simulink model "SimulinkModel_OWC_Array_Generator_Control_Varying_Theta"  (R2017b)
settings: Solver=ode4  StartTime=0.0  StopTime=tsim  FixedStep=delta_t  RelTol=1e-3
values from neighbouring files (symbols this model uses):
  a_gen = 0.0001    [InputDataExtraction.m]
  activate_HSSV = 1    [InputDataExtraction.m]
  Ainf_inv = inv(Ainf)    [InputDataExtraction.m]
  alpha1 = 219.4    [InputDataExtraction.m]
  alpha2 = 219.54    [InputDataExtraction.m]
  alpha3 = 219.4    [InputDataExtraction.m]
  B = zeros(vz,hz)    [ACTOR_CRITIC & SARSA.m]    (also in InputDataExtraction.m = 0.01; TDlearningExampleEforPosting.m)
  b_gen = 3.6    [InputDataExtraction.m]
  Beta = 30    [InputDataExtraction.m]
  d_t = 0.5    [InputDataExtraction.m]
  FEX = squeeze(FEX_ma_temp(:,ind_w-1+step)- ((omega -FEX_Sim.Omega(ind_w-1))/(FEX_Sim.Omega(ind_w)-FEX_Sim.Omega(ind_w-1))*(FEX_ma_temp(:,ind_w+step)-FEX_ma_temp(:,ind_w-1+step))))    [InputDataExtraction.m]
  FEX_ph = FEX_ph.*pi./180    [InputDataExtraction.m]
  gamma = 0.1    [CS533DQN_FunctionApproximation.m]    (also in ContinousControl.m = 0.75; DeepQLearningF.m = 0.25; HopeGreatRLCode.m = 0.3; InputDataExtraction.m = 1.4)
  h_zero = 15    [InputDataExtraction.m]
  Height = states_space(next_stPrimee_idx,1)    [ContinousControl.m]    (also in DeepQLearningF.m = states_space(state_idx,1); EtanStateExtraction.m = HeightVec(h); Forward_step.m = states_space( st_chosen,1); InputDataExtraction.m = HeightVec(h))
  I_c = [0 ... (first row only)    [InputDataExtraction.m]
  I_c_kin = [55 ... (first row only)    [InputDataExtraction.m]
  I_c_turb = [0 ... (first row only)    [InputDataExtraction.m]
  i_ms = 1.7    [InputDataExtraction.m]
  J = 3.06    [InputDataExtraction.m]
  K_buoancy = diag([ -rho*g*(S_b-S_p) -rho*g*(S_b-S_p) -rho*g*(S_b-S_p) -rho*g*S_p -rho*g*S_p -rho*g*S_p])    [InputDataExtraction.m]
  K_mooring = diag([K_m K_m K_m 0 0 0])    [InputDataExtraction.m]
  K_pressure = [ p_at*S_p p_at*S_p p_at*S_p]    [InputDataExtraction.m]
  L_m = 7.413    [InputDataExtraction.m]
  L_s = 0.13    [InputDataExtraction.m]
  Nt = 2    [InputDataExtraction.m]
  omega = (2*pi)/Ts    (= 0.628318530718)    [InputDataExtraction.m]
  OmegaStar = 6000/60    (= 100)    [InputDataExtraction.m]
  p_at = 1.01325*10e5    (= 1013250)    [InputDataExtraction.m]
  poles = 2    [InputDataExtraction.m]
  rho_at = 1.2041    [InputDataExtraction.m]
  s1 = 0.11    [InputDataExtraction.m]
  s2 = 0.11    [InputDataExtraction.m]
  s3 = 0.11    [InputDataExtraction.m]
  S_p = (d_p/2)^2*pi    (= 15.7632552987)    [InputDataExtraction.m]
  T_loss = 3    [InputDataExtraction.m]
  time_shift = -min(FEX_ph*Tp)*ones(6,1)    [InputDataExtraction.m]
  Tp = Ts    (= 10)    [InputDataExtraction.m]    (also in LetsStartIt.m = Ts; SafeLetsStartIt.m = Ts; StateExtraction.m = Ts)
  wave_delay = [wave_delay; wave_delay]    [InputDataExtraction.m]
undefined symbols (not defined in the file or in its folder): A_SS_R, B_SS_R, C_SS_R, D_SS_R
settings Model: Creator=danie  LastModifiedBy=browdani
settings OptimizationCC: LifeSpan=inf
settings DebuggingCC: SFExecutionAtInitializationDiag=none
settings CodeAppCC: StateflowObjectComments=on

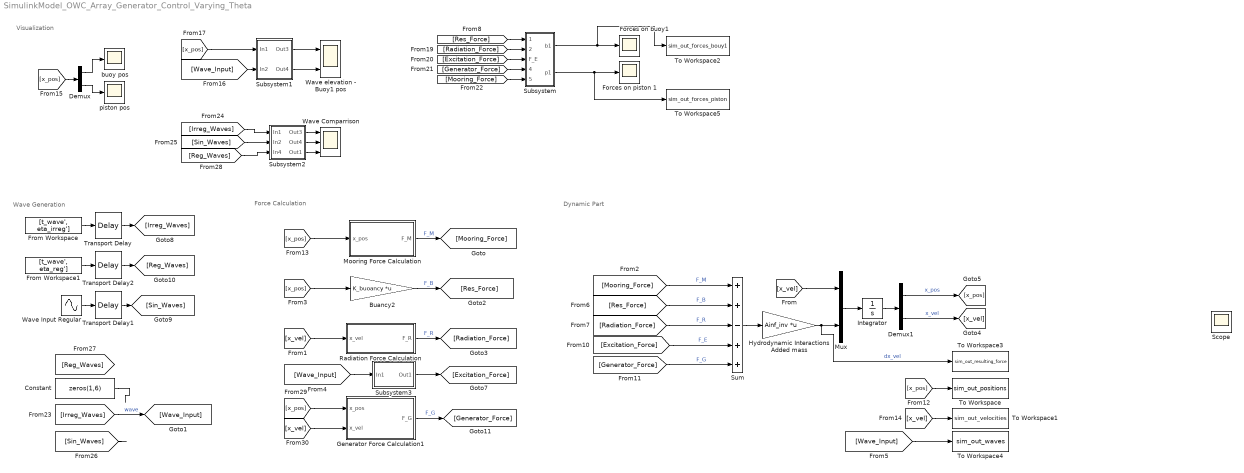
== system SimulinkModel_OWC_Array_Generator_Control_Varying_Theta ==
  note: Wave Generation
  note: Force Calculation
  note: Visualization
  note: Dynamic Part
  Buancy2 : Gain  Gain=K_buoancy  Multiplication=Matrix(K*u)
  Constant : Constant  Value=zeros(1,6)
  Demux : Demux  Outputs=2
  Demux1 : Demux  Outputs=2
  "Forces on buoy1 " : Scope
  Forces on piston 1 : Scope
  From Workspace : FromWorkspace  VariableName=[t_wave', eta_irreg']  SampleTime=0
  From Workspace1 : FromWorkspace  VariableName=[t_wave', eta_reg']  SampleTime=0
  Generator Force Calculation1 : Subsystem
  Hydrodynamic Interactions Added mass : Gain  Gain=Ainf_inv  Multiplication=Matrix(K*u)
  Integrator : Integrator  InitialCondition=I_c
  "Mooring Force Calculation " : Subsystem
  Mux : Mux  Inputs=2
  Radiation Force Calculation : Subsystem
  Subsystem : Subsystem
  Subsystem1 : Subsystem
  Subsystem2 : Subsystem
  Subsystem3 : Subsystem
  Sum : Sum  Inputs=++-++
  To Workspace : ToWorkspace  VariableName=sim_out_positions  SampleTime=-1
  To Workspace1 : ToWorkspace  VariableName=sim_out_velocities  SampleTime=-1
  To Workspace2 : ToWorkspace  VariableName=sim_out_forces_bouy1  SampleTime=-1
  To Workspace3 : ToWorkspace  VariableName=sim_out_resulting_force  SampleTime=-1
  To Workspace4 : ToWorkspace  VariableName=sim_out_waves  SampleTime=-1
  To Workspace5 : ToWorkspace  VariableName=sim_out_forces_piston  SampleTime=-1
  Transport Delay : TransportDelay  DelayTime=wave_delay +(time_shift+FEX_ph*Tp)
  Transport Delay1 : TransportDelay  DelayTime=wave_delay +(time_shift+FEX_ph*Tp)
  Transport Delay2 : TransportDelay  DelayTime=wave_delay +(time_shift+FEX_ph*Tp)
  Wave Comparrison : Scope  NumInputPorts=3
  Wave Input Regular : Sin  Amplitude=Height/2  Frequency=omega  Phase=FEX_ph  SampleTime=0
  "Wave elevation - Buoy1 pos " : Scope  NumInputPorts=2
  "buoy pos " : Scope
  "piston pos " : Scope
  Scope : Scope
  wires:
  [x_vel] -> Radiation Force Calculation/1(x_vel)
  Sum/1 -> Hydrodynamic Interactions Added mass/1
  Demux1/2 -> [x_vel]  "x_vel"
  Demux1/1 -> [x_pos]  "x_pos"
  Hydrodynamic Interactions Added mass/1 -> To Workspace3/1, Mux/2  "dx_vel"
  Subsystem/1(b1) -> To Workspace2/1, "Forces on buoy1 "/1
  Subsystem/2(p1) -> To Workspace5/1, Forces on piston 1/1
  [x_pos] -> "Mooring Force Calculation "/1(x_pos)
  [Generator_Force] -> Sum/5  "F_G"
  Subsystem1/1(Out3) -> "Wave elevation - Buoy1 pos "/1
  Subsystem1/2(Out4) -> "Wave elevation - Buoy1 pos "/2
  [Res_Force] -> Sum/2  "F_B"
  "Mooring Force Calculation "/1(F_M) -> [Mooring_Force]  "F_M"
  [Mooring_Force] -> Sum/1  "F_M"
  [Wave_Input] -> Subsystem3/1(In1)
  [x_pos] -> Buancy2/1
  Buancy2/1 -> [Res_Force]  "F_B"
  Radiation Force Calculation/1(F_R) -> [Radiation_Force]  "F_R"
  [Radiation_Force] -> Sum/3  "F_R"
  [Excitation_Force] -> Sum/4  "F_E"
  [x_pos] -> To Workspace/1
  [x_vel] -> To Workspace1/1
  [x_pos] -> Demux/1
  Demux/1 -> "buoy pos "/1
  Demux/2 -> "piston pos "/1
  [Wave_Input] -> Subsystem1/2(In2)
  [x_pos] -> Subsystem1/1(In1)
  [Res_Force] -> Subsystem/1(F_B)
  [Radiation_Force] -> Subsystem/2(F_R)
  [Excitation_Force] -> Subsystem/3(F_E)
  [Generator_Force] -> Subsystem/4(F_G)
  [Mooring_Force] -> Subsystem/5(F_M)
  Wave Input Regular/1 -> Transport Delay1/1
  [Irreg_Waves] -> Subsystem2/1(In1)
  [Sin_Waves] -> Subsystem2/2(In2)
  [Sin_Waves] -> ?
  Constant/1 -> ?
  From Workspace/1 -> Transport Delay/1
  Transport Delay/1 -> [Irreg_Waves]
  Transport Delay1/1 -> [Sin_Waves]
  Transport Delay2/1 -> [Reg_Waves]
  From Workspace1/1 -> Transport Delay2/1
  [Reg_Waves] -> Subsystem2/3(In4)
  Generator Force Calculation1/1(F_G) -> [Generator_Force]  "F_G"
  [x_vel] -> Generator Force Calculation1/2(x_vel)
  [x_pos] -> Generator Force Calculation1/1("x_pos ")
  [x_vel] -> Mux/1
  Mux/1 -> Integrator/1
  Integrator/1 -> Demux1/1
  Subsystem2/1(Out3) -> Wave Comparrison/1
  Subsystem2/2(Out4) -> Wave Comparrison/2
  Subsystem2/3(Out1) -> Wave Comparrison/3
  Subsystem3/1(Out1) -> [Excitation_Force]
  [Wave_Input] -> To Workspace4/1
  [Irreg_Waves] -> [Wave_Input]  "wave"

== system SimulinkModel_OWC_Array_Generator_Control_Varying_Theta/Generator Force Calculation1 ==
  "x_pos " : Inport
  x_vel : Inport  Port=2
  Gain : Gain  Gain=K_pressure
  Gain1 : Gain  Gain=-K_pressure
  Mux3 : Mux  Inputs=2
  To Workspace : ToWorkspace  VariableName=sim_out_chamber_pressure  SampleTime=-1
  Turbine/Generator Dynamics : Subsystem
  F_G : Outport
  wires:
  "x_pos "/1 -> Turbine/Generator Dynamics/1(x_pos)
  x_vel/1 -> Turbine/Generator Dynamics/2("x_vel ")
  Turbine/Generator Dynamics/1("p* ") -> Gain/1, Gain1/1, To Workspace/1
  Mux3/1 -> F_G/1  "F_G"
  Gain1/1 -> Mux3/2
  Gain/1 -> Mux3/1

== system SimulinkModel_OWC_Array_Generator_Control_Varying_Theta/Mooring Force Calculation  ==
  x_pos : Inport
  Buancy1 : Gain  Gain=K_mooring  Multiplication=Matrix(K*u)
  Constant : Constant  Value=0
  "Only if heave coordinte >0, extension of cables" : MinMax  Function=max  Inputs=2
  F_M : Outport
  wires:
  Constant/1 -> "Only if heave coordinte >0, extension of cables"/2
  Buancy1/1 -> F_M/1  "F_M"
  x_pos/1 -> "Only if heave coordinte >0, extension of cables"/1
  "Only if heave coordinte >0, extension of cables"/1 -> Buancy1/1

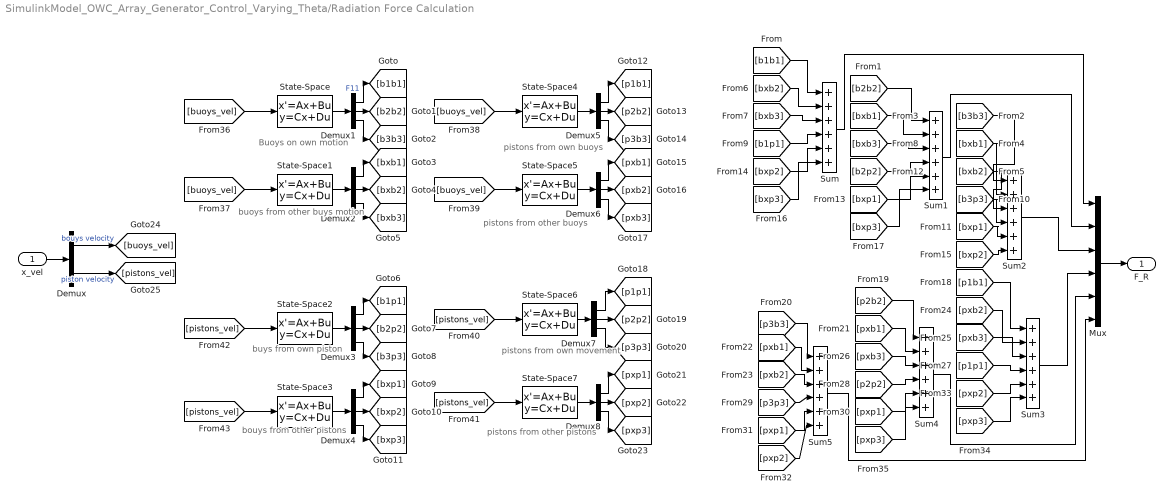
== system SimulinkModel_OWC_Array_Generator_Control_Varying_Theta/Radiation Force Calculation ==
  note: bouys from other pistons
  note: buys from own piston
  note: buoys from other buys motion
  note: Buoys on own motion
  note: pistons from other buoys
  note: pistons from own movement
  note: pistons from other pistons
  note: pistons from own buoys
  x_vel : Inport
  Demux : Demux  Outputs=2
  Demux{1..8} (8 alike) : Demux  Outputs=3
  Mux : Mux  Inputs=6
  State-Space : StateSpace  A=A_SS_R{1}  B=B_SS_R{1}  C=C_SS_R{1}  D=D_SS_R{1}  InitialCondition=0
  State-Space1 : StateSpace  A=A_SS_R{2}  B=B_SS_R{2}  C=C_SS_R{2}  D=D_SS_R{2}  InitialCondition=0
  State-Space2 : StateSpace  A=A_SS_R{3}  B=B_SS_R{3}  C=C_SS_R{3}  D=D_SS_R{3}  InitialCondition=0
  State-Space3 : StateSpace  A=A_SS_R{4}  B=B_SS_R{4}  C=C_SS_R{4}  D=D_SS_R{4}  InitialCondition=0
  State-Space4 : StateSpace  A=A_SS_R{5}  B=B_SS_R{5}  C=C_SS_R{5}  D=D_SS_R{5}  InitialCondition=0
  State-Space5 : StateSpace  A=A_SS_R{6}  B=B_SS_R{6}  C=C_SS_R{6}  D=D_SS_R{6}  InitialCondition=0
  State-Space6 : StateSpace  A=A_SS_R{7}  B=B_SS_R{7}  C=C_SS_R{7}  D=D_SS_R{7}  InitialCondition=0
  State-Space7 : StateSpace  A=A_SS_R{8}  B=B_SS_R{8}  C=C_SS_R{8}  D=D_SS_R{8}  InitialCondition=0
  Sum{,1..5} (6 alike) : Sum  Inputs=6
  F_R : Outport
  wires:
  Mux/1 -> F_R/1
  Sum/1 -> Mux/1
  State-Space/1 -> Demux1/1
  State-Space1/1 -> Demux2/1
  State-Space2/1 -> Demux3/1
  State-Space3/1 -> Demux4/1
  x_vel/1 -> Demux/1
  Sum2/1 -> Mux/3
  Sum3/1 -> Mux/4
  State-Space4/1 -> Demux5/1
  State-Space5/1 -> Demux6/1
  State-Space7/1 -> Demux8/1
  Sum4/1 -> Mux/5
  Sum5/1 -> Mux/6
  Demux1/1 -> [b1b1]  "F11"
  [b1b1] -> Sum/1
  Demux1/2 -> [b2b2]
  [b3b3] -> Sum2/1
  Demux1/3 -> [b3b3]
  Demux2/1 -> [bxb1]
  [bxb1] -> Sum1/2
  [b2b2] -> Sum1/1
  [bxb1] -> Sum2/2
  Demux2/2 -> [bxb2]
  [bxb2] -> Sum2/3
  Demux2/3 -> [bxb3]
  [bxb3] -> Sum/3
  [bxb3] -> Sum1/3
  Demux3/1 -> [b1p1]
  [b1p1] -> Sum/4
  Demux3/2 -> [b2p2]
  Demux3/3 -> [b3p3]
  [b3p3] -> Sum2/4
  Demux4/1 -> [bxp1]
  [bxp1] -> Sum2/5
  [b2p2] -> Sum1/4
  [bxp1] -> Sum1/5
  Demux4/2 -> [bxp2]
  [bxp2] -> Sum/5
  [bxp2] -> Sum2/6
  Demux4/3 -> [bxp3]
  [bxp3] -> Sum/6
  [bxp3] -> Sum1/6
  Sum1/1 -> Mux/2
  Demux5/1 -> [p1b1]
  [p1b1] -> Sum3/1
  Demux5/2 -> [p2b2]
  [p2b2] -> Sum4/1
  Demux5/3 -> [p3b3]
  [p3b3] -> Sum5/1
  Demux6/1 -> [pxb1]
  [pxb1] -> Sum4/2
  [pxb1] -> Sum5/2
  Demux6/2 -> [pxb2]
  [pxb2] -> Sum5/3
  [pxb2] -> Sum3/2
  Demux6/3 -> [pxb3]
  [pxb3] -> Sum3/3
  [pxb3] -> Sum4/3
  Demux7/1 -> [p1p1]
  [p1p1] -> Sum3/4
  Demux7/2 -> [p2p2]
  [p2p2] -> Sum4/4
  Demux7/3 -> [p3p3]
  [p3p3] -> Sum5/4
  Demux8/1 -> [pxp1]
  [pxp1] -> Sum4/5
  [pxp1] -> Sum5/5
  Demux8/2 -> [pxp2]
  [pxp2] -> Sum5/6
  [pxp2] -> Sum3/5
  Demux8/3 -> [pxp3]
  [pxp3] -> Sum3/6
  [pxp3] -> Sum4/6
  [buoys_vel] -> State-Space1/1
  [bxb2] -> Sum/2
  [pistons_vel] -> State-Space3/1
  [buoys_vel] -> State-Space5/1
  [pistons_vel] -> State-Space7/1
  State-Space6/1 -> Demux7/1
  Demux/1 -> [buoys_vel]  "bouys velocity"
  [buoys_vel] -> State-Space/1
  [buoys_vel] -> State-Space4/1
  Demux/2 -> [pistons_vel]  "piston velocity"
  [pistons_vel] -> State-Space6/1
  [pistons_vel] -> State-Space2/1

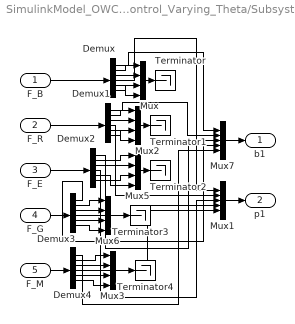
== system SimulinkModel_OWC_Array_Generator_Control_Varying_Theta/Subsystem ==
  F_B : Inport
  F_R : Inport  Port=2
  F_E : Inport  Port=3
  F_G : Inport  Port=4
  F_M : Inport  Port=5
  Demux{,1..4} (5 alike) : Demux  Outputs=6
  Mux{,2..3,5..6} (5 alike) : Mux
  Mux1 : Mux  Inputs=5
  Mux7 : Mux  Inputs=5
  Terminator{,1..4} (5 alike) : Terminator
  b1 : Outport
  p1 : Outport  Port=2
  wires:
  Demux3/1 -> Mux7/4
  Mux7/1 -> b1/1
  F_R/1 -> Demux1/1
  F_E/1 -> Demux2/1
  F_B/1 -> Demux/1
  F_G/1 -> Demux3/1
  Mux/1 -> Terminator/1
  Demux/1 -> Mux7/1
  Demux2/1 -> Mux7/3
  Demux1/1 -> Mux7/2
  Demux/3 -> Mux/2
  Demux/4 -> Mux1/1
  Demux/2 -> Mux/1
  Demux/5 -> Mux/4
  Demux/6 -> Mux/3
  Demux1/6 -> Mux2/3
  Demux1/3 -> Mux2/2
  Demux1/2 -> Mux2/1
  Mux2/1 -> Terminator1/1
  Demux1/5 -> Mux2/4
  Demux1/4 -> Mux1/2
  Demux3/2 -> Mux6/1
  Demux2/3 -> Mux5/2
  Mux6/1 -> Terminator3/1
  Demux2/2 -> Mux5/1
  Demux3/6 -> Mux6/4
  Demux2/4 -> Mux1/3
  Demux3/3 -> Mux6/2
  Demux3/4 -> Mux1/4
  Mux5/1 -> Terminator2/1
  Demux2/5 -> Mux5/4
  Demux3/5 -> Mux6/3
  Demux2/6 -> Mux5/3
  Mux1/1 -> p1/1
  F_M/1 -> Demux4/1
  Demux4/1 -> Mux7/5
  Demux4/4 -> Mux1/5
  Demux4/2 -> Mux3/1
  Demux4/3 -> Mux3/2
  Demux4/5 -> Mux3/3
  Demux4/6 -> Mux3/4
  Mux3/1 -> Terminator4/1

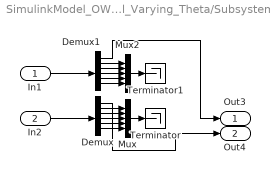
== system SimulinkModel_OWC_Array_Generator_Control_Varying_Theta/Subsystem1 ==
  In1 : Inport
  In2 : Inport  Port=2
  Demux : Demux  Outputs=6
  Demux1 : Demux  Outputs=6
  Mux : Mux  Inputs=5
  Mux2 : Mux  Inputs=5
  Terminator : Terminator
  Terminator1 : Terminator
  Out3 : Outport
  Out4 : Outport  Port=2
  wires:
  Demux1/2 -> Mux2/1
  Demux1/3 -> Mux2/2
  Mux2/1 -> Terminator1/1
  Mux/1 -> Terminator/1
  In1/1 -> Demux1/1
  In2/1 -> Demux/1
  Demux1/5 -> Mux2/4
  Demux1/6 -> Mux2/5
  Demux1/4 -> Mux2/3
  Demux/1 -> Out4/1
  Demux/2 -> Mux/1
  Demux/3 -> Mux/2
  Demux/4 -> Mux/3
  Demux/6 -> Mux/5
  Demux/5 -> Mux/4
  Demux1/1 -> Out3/1

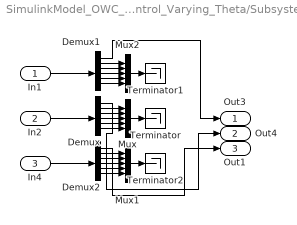
== system SimulinkModel_OWC_Array_Generator_Control_Varying_Theta/Subsystem2 ==
  In1 : Inport
  In2 : Inport  Port=2
  In4 : Inport  Port=3
  Demux : Demux  Outputs=6
  Demux1 : Demux  Outputs=6
  Demux2 : Demux  Outputs=6
  Mux : Mux  Inputs=5
  Mux1 : Mux  Inputs=5
  Mux2 : Mux  Inputs=5
  Terminator : Terminator
  Terminator1 : Terminator
  Terminator2 : Terminator
  Out3 : Outport
  Out4 : Outport  Port=2
  Out1 : Outport  Port=3
  wires:
  Demux1/1 -> Out3/1
  Demux/5 -> Mux/4
  Demux/6 -> Mux/5
  Demux/4 -> Mux/3
  Demux/3 -> Mux/2
  Demux/2 -> Mux/1
  Demux/1 -> Out4/1
  Demux1/4 -> Mux2/3
  Demux1/6 -> Mux2/5
  Demux1/5 -> Mux2/4
  In2/1 -> Demux/1
  In1/1 -> Demux1/1
  Mux/1 -> Terminator/1
  Mux2/1 -> Terminator1/1
  Demux1/3 -> Mux2/2
  Demux1/2 -> Mux2/1
  Mux1/1 -> Terminator2/1
  In4/1 -> Demux2/1
  Demux2/1 -> Out1/1
  Demux2/2 -> Mux1/1
  Demux2/3 -> Mux1/2
  Demux2/4 -> Mux1/3
  Demux2/6 -> Mux1/5
  Demux2/5 -> Mux1/4

== system SimulinkModel_OWC_Array_Generator_Control_Varying_Theta/Subsystem3 ==
  In1 : Inport
  "Check if user input equals irregular waves, then the special irregular excitation force, else the user input times the linear excitation force coeff" : MATLAB Function  TreatAsAtomicUnit=on
  Constant : Constant
  From Workspace1 : FromWorkspace  VariableName=[t_wave', eta_irreg']  SampleTime=0
  From Workspace4 : FromWorkspace  VariableName=[t_wave', Fex_irreg']  SampleTime=0
  Gain1 : Gain  Gain=FEX
  Transport Delay1 : TransportDelay  DelayTime=wave_delay +(time_shift+FEX_ph*Tp)
  Out1 : Outport
  wires:
  In1/1 -> "Check if user input equals irregular waves, then the special irregular excitation force, else the user input times the linear excitation force coeff"/1(userWaves)
  From Workspace1/1 -> Transport Delay1/1
  From Workspace4/1 -> "Check if user input equals irregular waves, then the special irregular excitation force, else the user input times the linear excitation force coeff"/3(irregEx)
  "Check if user input equals irregular waves, then the special irregular excitation force, else the user input times the linear excitation force coeff"/1(y) -> Out1/1
  Gain1/1 -> "Check if user input equals irregular waves, then the special irregular excitation force, else the user input times the linear excitation force coeff"/4(FEX)
  Constant/1 -> Gain1/1
  Transport Delay1/1 -> "Check if user input equals irregular waves, then the special irregular excitation force, else the user input times the linear excitation force coeff"/2(irregEta)

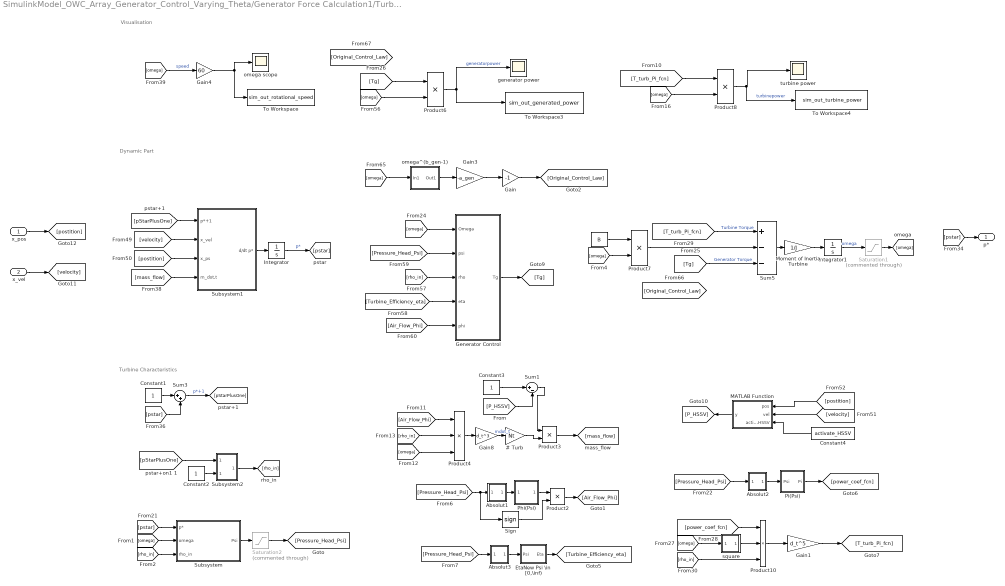
== system SimulinkModel_OWC_Array_Generator_Control_Varying_Theta/Generator Force Calculation1/Turbine//Generator Dynamics ==
  note: Dynamic Part
  note: Visualisation
  note: Turbine Characteristics
  x_pos : Inport
  "x_vel " : Inport  Port=2
  " " : Constant  Value=B
  # Turb : Gain  Gain=Nt
  Absolut1 : Subsystem
  Absolut2 : Subsystem
  Absolut3 : Subsystem
  Constant1 : Constant
  Constant2 : Constant
  Constant3 : Constant
  Constant4 : Constant  Value=activate_HSSV
  EtaNew Psi \in [0,\inf) : Subsystem
  Gain : Gain  Gain=-1
  Gain1 : Gain  Gain=d_t^5
  Gain3 : Gain  Gain=-a_gen
  Gain4 : Gain  Gain=60
  Gain8 : Gain  Gain=d_t^3
  Generator Control : Subsystem
  Integrator : Integrator  InitialCondition=I_c_turb
  Integrator1 : Integrator  InitialCondition=I_c_kin
  MATLAB Function : MATLAB Function  TreatAsAtomicUnit=on
  Moment of Inertia Turbine : Gain  Gain=1/J
  "Phi(Psi) " : Subsystem
  Pi(Psi) : Subsystem
  Product10 : Product  Inputs=***
  Product2 : Product
  Product3 : Product
  Product4 : Product  Inputs=***
  Product6 : Product  Inputs=**
  Product7 : Product  Inputs=**
  Product8 : Product  Inputs=**
  Saturation1 : Saturate  Commented=through  UpperLimit=120  LowerLimit=20
  Saturation2 : Saturate  Commented=through  UpperLimit=8  LowerLimit=-8
  Sign : Signum
  Subsystem : Subsystem
  Subsystem1 : Subsystem
  Subsystem2 : Subsystem
  Sum1 : Sum  Inputs=|+-
  Sum3 : Sum  Inputs=|++
  Sum5 : Sum  Inputs=+--
  To Workspace : ToWorkspace  VariableName=sim_out_rotational_speed  SampleTime=-1
  To Workspace3 : ToWorkspace  VariableName=sim_out_generated_power  SampleTime=-1
  To Workspace4 : ToWorkspace  VariableName=sim_out_turbine_power  SampleTime=-1
  generator power : Scope
  "omega scope " : Scope
  omega^(b_gen-1) : Subsystem
  "square " : Subsystem
  turbine power : Scope
  "p* " : Outport
  wires:
  Moment of Inertia Turbine/1 -> Integrator1/1
  "Phi(Psi) "/1(Out1) -> Product2/1
  Subsystem1/1(d/dt p*) -> Integrator/1
  [mass_flow] -> Subsystem1/4(m_dot,t)
  x_pos/1 -> [postition]
  "x_vel "/1 -> [velocity]
  [pStarPlusOne] -> Subsystem1/1(p*+1)
  Gain8/1 -> # Turb/1  "mdot_t"
  [pstar] -> Sum3/2
  [pstar] -> "p* "/1
  Gain1/1 -> [T_turb_Pi_fcn]
  [rho_in] -> Product10/3
  "square "/1(Out1) -> Product10/2
  [omega] -> "square "/1(In1)
  [power_coef_fcn] -> Product10/1
  Product10/1 -> Gain1/1
  Pi(Psi)/1(Pi) -> [power_coef_fcn]
  [Pressure_Head_Psi] -> Absolut2/1(In1)
  Absolut2/1(Out1) -> Pi(Psi)/1(Psi)
  Sign/1 -> Product2/2
  Absolut1/1(Out1) -> "Phi(Psi) "/1(In1)
  Constant2/1 -> Subsystem2/2(1)
  [pStarPlusOne] -> Subsystem2/1(p*+1)
  Subsystem2/1(rho_in) -> [rho_in]
  [Pressure_Head_Psi] -> Absolut1/1(In1), Sign/1
  [rho_in] -> Subsystem/3(rho_in)
  [omega] -> Subsystem/2(omega)
  [pstar] -> Subsystem/1(p*)
  Subsystem/1(Psi) -> Saturation2/1
  Product4/1 -> Gain8/1
  [omega] -> Product4/3
  [rho_in] -> Product4/2
  [Air_Flow_Phi] -> Product4/1
  Integrator1/1 -> Saturation1/1  "omega"
  Sum3/1 -> [pStarPlusOne]  "p*+1"
  Integrator/1 -> [pstar]  "p*"
  Constant1/1 -> Sum3/1
  EtaNew Psi \in [0,\inf)/1(Eta) -> [Turbine_Efficiency_eta]
  [Pressure_Head_Psi] -> Absolut3/1(In1)
  Absolut3/1(Out1) -> EtaNew Psi \in [0,\inf)/1(Psi)
  Product2/1 -> [Air_Flow_Phi]
  Saturation1/1 -> [omega]
  Saturation2/1 -> [Pressure_Head_Psi]
  # Turb/1 -> Product3/2
  Product3/1 -> [mass_flow]
  [P_HSSV] -> Sum1/2
  [velocity] -> Subsystem1/2("x_vel ")
  [postition] -> Subsystem1/3(x_ps)
  MATLAB Function/1(y) -> [P_HSSV]
  [postition] -> MATLAB Function/1(pos)
  [velocity] -> MATLAB Function/2(vel)
  Constant3/1 -> Sum1/1
  Sum1/1 -> Product3/1
  Constant4/1 -> MATLAB Function/3(activate_HSSV)
  [omega] -> Product6/2
  Product6/1 -> To Workspace3/1, generator power/1  "generatorpower"
  [omega] -> Generator Control/1(Omega)
  Generator Control/1(Tg) -> [Tg]
  Sum5/1 -> Moment of Inertia Turbine/1
  [T_turb_Pi_fcn] -> Sum5/1  "Turbine Torque"
  [Air_Flow_Phi] -> Generator Control/5(phi)
  [Turbine_Efficiency_eta] -> Generator Control/4(eta)
  [rho_in] -> Generator Control/3(rho)
  [Pressure_Head_Psi] -> Generator Control/2(psi)
  [omega] -> omega^(b_gen-1)/1(In1)
  omega^(b_gen-1)/1(Out1) -> Gain3/1
  [omega] -> Product7/2
  " "/1 -> Product7/1
  Product7/1 -> Sum5/2
  [omega] -> Product8/2
  [T_turb_Pi_fcn] -> Product8/1
  Product8/1 -> To Workspace4/1, turbine power/1  "turbinepower"
  Gain3/1 -> Gain/1
  Gain/1 -> [Original_Control_Law]
  Gain4/1 -> To Workspace/1, "omega scope "/1
  [omega] -> Gain4/1  "speed"
  [Tg] -> Product6/1
  [Tg] -> Sum5/3  "Generator Torque"

== system SimulinkModel_OWC_Array_Generator_Control_Varying_Theta/Generator Force Calculation1/Turbine//Generator Dynamics/Absolut1 ==
  In1 : Inport
  Abs : Abs
  Abs1 : Abs
  Abs2 : Abs
  Demux1 : Demux  Outputs=3
  Mux1 : Mux  Inputs=3
  Out1 : Outport
  wires:
  Mux1/1 -> Out1/1
  Demux1/3 -> Abs2/1
  Demux1/1 -> Abs/1
  Abs/1 -> Mux1/1
  Demux1/2 -> Abs1/1
  Abs1/1 -> Mux1/2
  Abs2/1 -> Mux1/3
  In1/1 -> Demux1/1

== system SimulinkModel_OWC_Array_Generator_Control_Varying_Theta/Generator Force Calculation1/Turbine//Generator Dynamics/Absolut2 ==
  In1 : Inport
  Abs : Abs
  Abs1 : Abs
  Abs2 : Abs
  Demux1 : Demux  Outputs=3
  Mux1 : Mux  Inputs=3
  Out1 : Outport
  wires:
  Mux1/1 -> Out1/1
  Demux1/3 -> Abs2/1
  Demux1/1 -> Abs/1
  Abs/1 -> Mux1/1
  Demux1/2 -> Abs1/1
  Abs1/1 -> Mux1/2
  Abs2/1 -> Mux1/3
  In1/1 -> Demux1/1

== system SimulinkModel_OWC_Array_Generator_Control_Varying_Theta/Generator Force Calculation1/Turbine//Generator Dynamics/Absolut3 ==
  In1 : Inport
  Abs : Abs
  Abs1 : Abs
  Abs2 : Abs
  Demux1 : Demux  Outputs=3
  Mux1 : Mux  Inputs=3
  Out1 : Outport
  wires:
  Mux1/1 -> Out1/1
  Demux1/3 -> Abs2/1
  Demux1/1 -> Abs/1
  Abs/1 -> Mux1/1
  Demux1/2 -> Abs1/1
  Abs1/1 -> Mux1/2
  Abs2/1 -> Mux1/3
  In1/1 -> Demux1/1

== system SimulinkModel_OWC_Array_Generator_Control_Varying_Theta/Generator Force Calculation1/Turbine//Generator Dynamics/EtaNew Psi \in [0,\inf) ==
  Psi : Inport
  Demux2 : Demux  Outputs=3
  Eta(Psi) : Fcn  Expr=(-1540*u^3 +22270*u^2 + 1631*u - 394.8)/(u^4 +1294*u^3 + 34120*u^2 -3081*u +491.6)
  Eta(Psi)1 : Fcn  Expr=(-1540*u^3 +22270*u^2 + 1631*u - 394.8)/(u^4 +1294*u^3 + 34120*u^2 -3081*u +491.6)
  Eta(Psi)2 : Fcn  Expr=(-1540*u^3 +22270*u^2 + 1631*u - 394.8)/(u^4 +1294*u^3 + 34120*u^2 -3081*u +491.6)
  Mux2 : Mux  Inputs=3
  Eta : Outport
  wires:
  Mux2/1 -> Eta/1
  Demux2/1 -> Eta(Psi)/1
  Demux2/3 -> Eta(Psi)2/1
  Eta(Psi)2/1 -> Mux2/3
  Demux2/2 -> Eta(Psi)1/1
  Eta(Psi)1/1 -> Mux2/2
  Eta(Psi)/1 -> Mux2/1
  Psi/1 -> Demux2/1

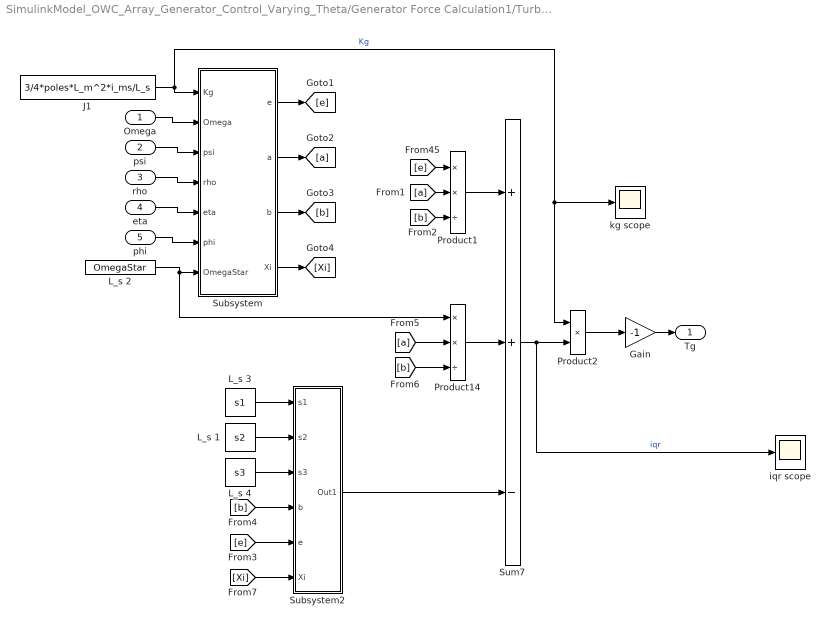
== system SimulinkModel_OWC_Array_Generator_Control_Varying_Theta/Generator Force Calculation1/Turbine//Generator Dynamics/Generator Control ==
  Omega : Inport
  psi : Inport  Port=2
  rho : Inport  Port=3
  eta : Inport  Port=4
  phi : Inport  Port=5
  Gain : Gain  Gain=-1
  J1 : Constant  Value=3/4*poles*L_m^2*i_ms/L_s
  L_s 1 : Constant  Value=s2
  L_s 2 : Constant  Value=OmegaStar
  L_s 3 : Constant  Value=s1
  L_s 4 : Constant  Value=s3
  Product1 : Product  Inputs=**/
  Product14 : Product  Inputs=**/
  Product2 : Product  Inputs=**
  Subsystem : Subsystem
  Subsystem2 : Subsystem
  Sum7 : Sum  Inputs=++-
  "iqr scope " : Scope
  kg scope : Scope
  Tg : Outport
  wires:
  Product14/1 -> Sum7/2
  Product1/1 -> Sum7/1
  Sum7/1 -> "iqr scope "/1, Product2/2  "iqr"
  J1/1 -> Subsystem/1(Kg), kg scope/1, Product2/1  "Kg"
  psi/1 -> Subsystem/3(psi)
  rho/1 -> Subsystem/4(rho)
  eta/1 -> Subsystem/5(eta)
  phi/1 -> Subsystem/6(phi)
  L_s 2/1 -> Product14/1, Subsystem/7(OmegaStar)
  Omega/1 -> Subsystem/2(Omega)
  Subsystem/4(Xi) -> [Xi]
  [e] -> Product1/1
  [a] -> Product1/2
  [a] -> Product14/2
  [b] -> Product1/3
  [b] -> Product14/3
  Subsystem/1(e) -> [e]
  Subsystem/2(a) -> [a]
  Subsystem/3(b) -> [b]
  Product2/1 -> Gain/1
  Gain/1 -> Tg/1
  L_s 3/1 -> Subsystem2/1(s1)
  L_s 1/1 -> Subsystem2/2(s2)
  L_s 4/1 -> Subsystem2/3(s3)
  [e] -> Subsystem2/5(e)
  [b] -> Subsystem2/4(b)
  [Xi] -> Subsystem2/6(Xi)
  Subsystem2/1(Out1) -> Sum7/3

== system SimulinkModel_OWC_Array_Generator_Control_Varying_Theta/Generator Force Calculation1/Turbine//Generator Dynamics/Phi(Psi)  ==
  In1 : Inport
  Demux1 : Demux  Outputs=3
  Mux1 : Mux  Inputs=3
  Phi(Psi) : Fcn  Expr=u^(1/1.724)*0.196
  Phi(Psi)1 : Fcn  Expr=u^(1/1.724)*0.196
  Phi(Psi)2 : Fcn  Expr=u^(1/1.724)*0.196
  Out1 : Outport
  wires:
  Phi(Psi)1/1 -> Mux1/1
  Phi(Psi)/1 -> Mux1/2
  Phi(Psi)2/1 -> Mux1/3
  Mux1/1 -> Out1/1
  Demux1/1 -> Phi(Psi)1/1
  Demux1/3 -> Phi(Psi)2/1
  Demux1/2 -> Phi(Psi)/1
  In1/1 -> Demux1/1

== system SimulinkModel_OWC_Array_Generator_Control_Varying_Theta/Generator Force Calculation1/Turbine//Generator Dynamics/Pi(Psi) ==
  Psi : Inport
  Demux2 : Demux  Outputs=3
  Mux2 : Mux  Inputs=3
  Pi(Psi) : Fcn  Expr=0.0003527*u^4 -0.008503*u^3 + 0.0525*u^2 +0.09456*u -0.007476
  Pi(Psi)1 : Fcn  Expr=0.0003527*u^4 -0.008503*u^3 + 0.0525*u^2 +0.09456*u -0.007476
  Pi(Psi)2 : Fcn  Expr=0.0003527*u^4 -0.008503*u^3 + 0.0525*u^2 +0.09456*u -0.007476
  Pi : Outport
  wires:
  Mux2/1 -> Pi/1
  Demux2/1 -> Pi(Psi)/1
  Demux2/3 -> Pi(Psi)2/1
  Pi(Psi)2/1 -> Mux2/3
  Demux2/2 -> Pi(Psi)1/1
  Pi(Psi)1/1 -> Mux2/2
  Pi(Psi)/1 -> Mux2/1
  Psi/1 -> Demux2/1

== system SimulinkModel_OWC_Array_Generator_Control_Varying_Theta/Generator Force Calculation1/Turbine//Generator Dynamics/Subsystem ==
  p* : Inport
  omega : Inport  Port=2
  rho_in : Inport  Port=3
  Gain5 : Gain  Gain=p_at/(d_t^2)
  Product2 : Product  Inputs=*//
  square : Subsystem
  Psi : Outport
  wires:
  square/1(Out1) -> Product2/2
  omega/1 -> square/1(In1)
  p*/1 -> Product2/1
  rho_in/1 -> Product2/3
  Product2/1 -> Gain5/1
  Gain5/1 -> Psi/1

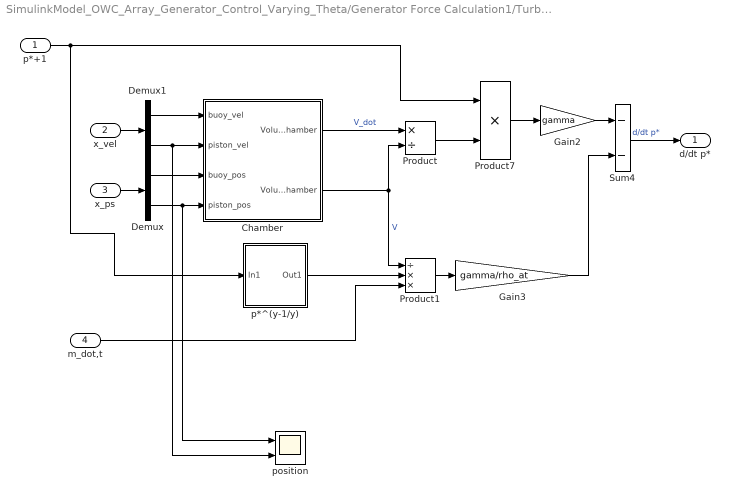
== system SimulinkModel_OWC_Array_Generator_Control_Varying_Theta/Generator Force Calculation1/Turbine//Generator Dynamics/Subsystem1 ==
  p*+1 : Inport
  "x_vel " : Inport  Port=2
  x_ps : Inport  Port=3
  m_dot,t : Inport  Port=4
  "Chamber " : Subsystem
  Demux : Demux  Outputs=2
  Demux1 : Demux  Outputs=2
  Gain2 : Gain  Gain=gamma
  Gain3 : Gain  Gain=gamma/rho_at
  Product : Product  Inputs=*/
  Product1 : Product  Inputs=/**
  Product7 : Product  Inputs=**
  Sum4 : Sum  Inputs=--
  p*^(y-1/y) : Subsystem
  position : Scope  NumInputPorts=2
  d/dt p* : Outport
  wires:
  m_dot,t/1 -> Product1/3
  Demux/2 -> position/1, "Chamber "/4("piston_pos ")
  x_ps/1 -> Demux/1
  Demux1/2 -> position/2, "Chamber "/2(piston_vel)
  "x_vel "/1 -> Demux1/1
  Demux/1 -> "Chamber "/3(buoy_pos)
  Demux1/1 -> "Chamber "/1(buoy_vel)
  "Chamber "/2(Volume Chamber) -> Product1/1, Product/2  "V"
  p*^(y-1/y)/1(Out1) -> Product1/2
  "Chamber "/1("Volume Change Chamber ") -> Product/1  "V_dot"
  Product7/1 -> Gain2/1
  Product1/1 -> Gain3/1
  Gain2/1 -> Sum4/1
  p*+1/1 -> Product7/1, p*^(y-1/y)/1(In1)
  Product/1 -> Product7/2
  Sum4/1 -> d/dt p*/1  "d/dt p*"
  Gain3/1 -> Sum4/2

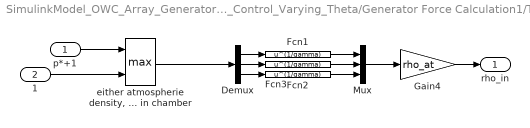
== system SimulinkModel_OWC_Array_Generator_Control_Varying_Theta/Generator Force Calculation1/Turbine//Generator Dynamics/Subsystem2 ==
  p*+1 : Inport
  1 : Inport  Port=2
  Demux : Demux  Outputs=3
  Fcn1 : Fcn  Expr=u^(1/gamma)
  Fcn2 : Fcn  Expr=u^(1/gamma)
  Fcn3 : Fcn  Expr=u^(1/gamma)
  Gain4 : Gain  Gain=rho_at
  Mux : Mux  Inputs=3
  "either atmospherie density, or pressure dependent density in chamber" : MinMax  Function=max  Inputs=2
  rho_in : Outport
  wires:
  Mux/1 -> Gain4/1
  Fcn1/1 -> Mux/1
  Demux/3 -> Fcn3/1
  Fcn3/1 -> Mux/3
  Fcn2/1 -> Mux/2
  Demux/2 -> Fcn2/1
  Demux/1 -> Fcn1/1
  "either atmospherie density, or pressure dependent density in chamber"/1 -> Demux/1
  p*+1/1 -> "either atmospherie density, or pressure dependent density in chamber"/1
  1/1 -> "either atmospherie density, or pressure dependent density in chamber"/2
  Gain4/1 -> rho_in/1

== system SimulinkModel_OWC_Array_Generator_Control_Varying_Theta/Generator Force Calculation1/Turbine//Generator Dynamics/omega^(b_gen-1) ==
  In1 : Inport
  Demux3 : Demux  Outputs=3
  Fcn1 : Fcn  Expr=u^(b_gen-1)
  Fcn2 : Fcn  Expr=u^(b_gen-1)
  Fcn3 : Fcn  Expr=u^(b_gen-1)
  Mux3 : Mux  Inputs=3
  Out1 : Outport
  wires:
  In1/1 -> Demux3/1
  Fcn1/1 -> Mux3/1
  Fcn3/1 -> Mux3/3
  Mux3/1 -> Out1/1
  Demux3/2 -> Fcn2/1
  Fcn2/1 -> Mux3/2
  Demux3/1 -> Fcn1/1
  Demux3/3 -> Fcn3/1

== system SimulinkModel_OWC_Array_Generator_Control_Varying_Theta/Generator Force Calculation1/Turbine//Generator Dynamics/square  ==
  In1 : Inport
  Demux1 : Demux  Outputs=3
  Math Function4 : Math  Operator=square  SaturateOnIntegerOverflow=on
  Math Function5 : Math  Operator=square  SaturateOnIntegerOverflow=on
  Math Function6 : Math  Operator=square  SaturateOnIntegerOverflow=on
  Mux1 : Mux  Inputs=3
  Out1 : Outport
  wires:
  Math Function6/1 -> Mux1/3
  Math Function4/1 -> Mux1/1
  Mux1/1 -> Out1/1
  Demux1/2 -> Math Function5/1
  Demux1/1 -> Math Function4/1
  In1/1 -> Demux1/1
  Demux1/3 -> Math Function6/1
  Math Function5/1 -> Mux1/2

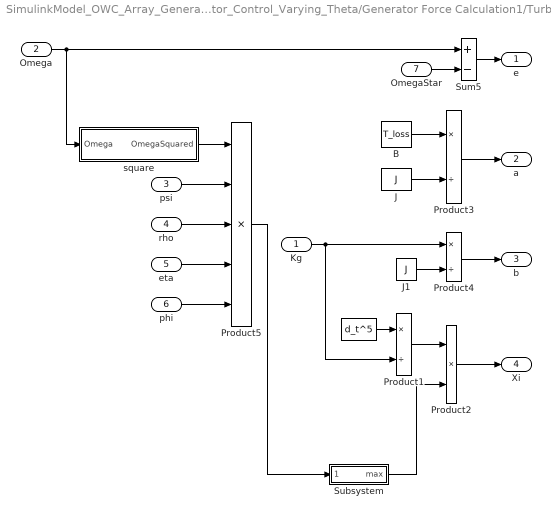
== system SimulinkModel_OWC_Array_Generator_Control_Varying_Theta/Generator Force Calculation1/Turbine//Generator Dynamics/Generator Control/Subsystem ==
  Kg : Inport
  Omega : Inport  Port=2
  psi : Inport  Port=3
  rho : Inport  Port=4
  eta : Inport  Port=5
  phi : Inport  Port=6
  OmegaStar : Inport  Port=7
  " " : Constant  Value=d_t^5
  "B " : Constant  Value=T_loss
  J : Constant  Value=J
  J1 : Constant  Value=J
  Product1 : Product  Inputs=*/
  Product2 : Product  Inputs=**
  Product3 : Product  Inputs=*/
  Product4 : Product  Inputs=*/
  Product5 : Product  Inputs=*****
  Subsystem : Subsystem
  Sum5 : Sum  Inputs=+-
  square : Subsystem
  e : Outport
  a : Outport  Port=2
  b : Outport  Port=3
  Xi : Outport  Port=4
  wires:
  "B "/1 -> Product3/1
  Product3/1 -> a/1
  J1/1 -> Product4/2
  Product4/1 -> b/1
  Sum5/1 -> e/1
  J/1 -> Product3/2
  OmegaStar/1 -> Sum5/2
  " "/1 -> Product1/1
  Product1/1 -> Product2/1
  Subsystem/1("max ") -> Product2/2
  Product2/1 -> Xi/1
  phi/1 -> Product5/5
  eta/1 -> Product5/4
  rho/1 -> Product5/3
  psi/1 -> Product5/2
  square/1("OmegaSquared ") -> Product5/1
  Product5/1 -> Subsystem/1(input2)
  Kg/1 -> Product1/2, Product4/1
  Omega/1 -> Sum5/1, square/1(Omega)

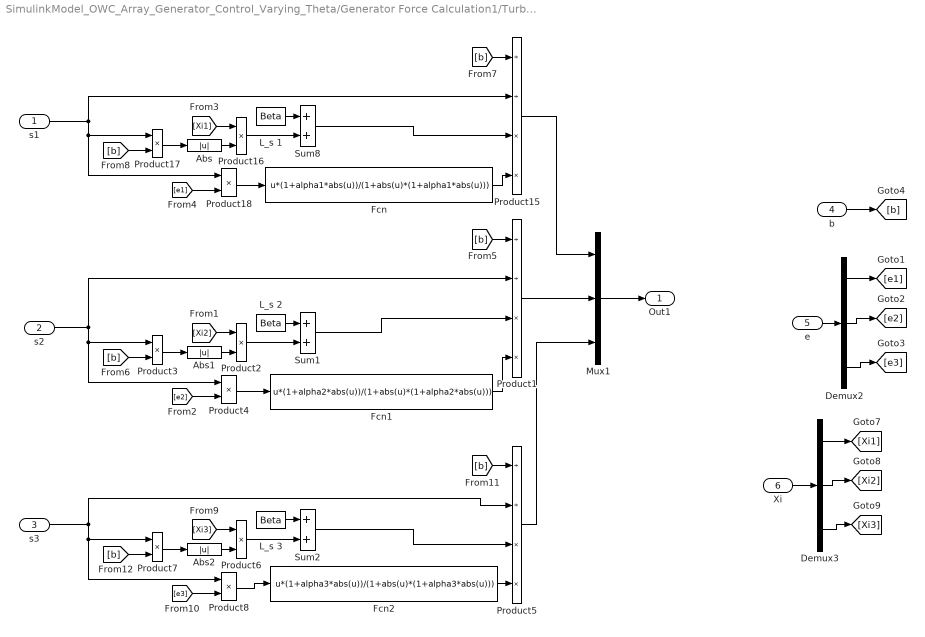
== system SimulinkModel_OWC_Array_Generator_Control_Varying_Theta/Generator Force Calculation1/Turbine//Generator Dynamics/Generator Control/Subsystem2 ==
  s1 : Inport
  s2 : Inport  Port=2
  s3 : Inport  Port=3
  b : Inport  Port=4
  e : Inport  Port=5
  Xi : Inport  Port=6
  Abs : Abs
  Abs1 : Abs
  Abs2 : Abs
  Demux2 : Demux  Outputs=3
  Demux3 : Demux  Outputs=3
  Fcn : Fcn  Expr=u*(1+alpha1*abs(u))/(1+abs(u)*(1+alpha1*abs(u)))
  Fcn1 : Fcn  Expr=u*(1+alpha2*abs(u))/(1+abs(u)*(1+alpha2*abs(u)))
  Fcn2 : Fcn  Expr=u*(1+alpha3*abs(u))/(1+abs(u)*(1+alpha3*abs(u)))
  L_s 1 : Constant  Value=Beta
  L_s 2 : Constant  Value=Beta
  L_s 3 : Constant  Value=Beta
  Mux1 : Mux  Inputs=3
  Product1 : Product  Inputs=//**
  Product15 : Product  Inputs=//**
  Product{2..4,6..8,16..18} (9 alike) : Product  Inputs=**
  Product5 : Product  Inputs=//**
  Sum1 : Sum
  Sum2 : Sum
  Sum8 : Sum
  Out1 : Outport
  wires:
  Product16/1 -> Sum8/2
  Product18/1 -> Fcn/1
  Product15/1 -> Mux1/1
  [Xi1] -> Product16/1
  Product17/1 -> Abs/1
  L_s 1/1 -> Sum8/1
  Fcn/1 -> Product15/4
  [e1] -> Product18/2
  [b] -> Product15/1
  [b] -> Product17/2
  s1/1 -> Product15/2, Product18/1, Product17/1
  Sum8/1 -> Product15/3
  Abs/1 -> Product16/2
  s2/1 -> Product1/2, Product4/1, Product3/1
  Abs1/1 -> Product2/2
  Sum1/1 -> Product1/3
  [b] -> Product1/1
  Product3/1 -> Abs1/1
  [b] -> Product3/2
  [Xi2] -> Product2/1
  Product1/1 -> Mux1/2
  L_s 2/1 -> Sum1/1
  Product2/1 -> Sum1/2
  [e2] -> Product4/2
  s3/1 -> Product5/2, Product8/1, Product7/1
  Abs2/1 -> Product6/2
  Sum2/1 -> Product5/3
  [b] -> Product5/1
  Product7/1 -> Abs2/1
  [b] -> Product7/2
  [Xi3] -> Product6/1
  Product5/1 -> Mux1/3
  L_s 3/1 -> Sum2/1
  Product6/1 -> Sum2/2
  [e3] -> Product8/2
  e/1 -> Demux2/1
  Demux2/1 -> [e1]
  Demux2/2 -> [e2]
  Demux2/3 -> [e3]
  Demux3/1 -> [Xi1]
  Demux3/3 -> [Xi3]
  Demux3/2 -> [Xi2]
  Xi/1 -> Demux3/1
  Mux1/1 -> Out1/1
  Product4/1 -> Fcn1/1
  Fcn1/1 -> Product1/4
  Fcn2/1 -> Product5/4
  Product8/1 -> Fcn2/1
  b/1 -> [b]

== system SimulinkModel_OWC_Array_Generator_Control_Varying_Theta/Generator Force Calculation1/Turbine//Generator Dynamics/Subsystem/square ==
  In1 : Inport
  Demux5 : Demux  Outputs=3
  Math Function4 : Math  Operator=square  SaturateOnIntegerOverflow=on
  Math Function5 : Math  Operator=square  SaturateOnIntegerOverflow=on
  Math Function6 : Math  Operator=square  SaturateOnIntegerOverflow=on
  Mux5 : Mux  Inputs=3
  Out1 : Outport
  wires:
  Demux5/3 -> Math Function6/1
  Demux5/1 -> Math Function4/1
  Math Function5/1 -> Mux5/2
  Math Function4/1 -> Mux5/1
  Math Function6/1 -> Mux5/3
  In1/1 -> Demux5/1
  Mux5/1 -> Out1/1
  Demux5/2 -> Math Function5/1

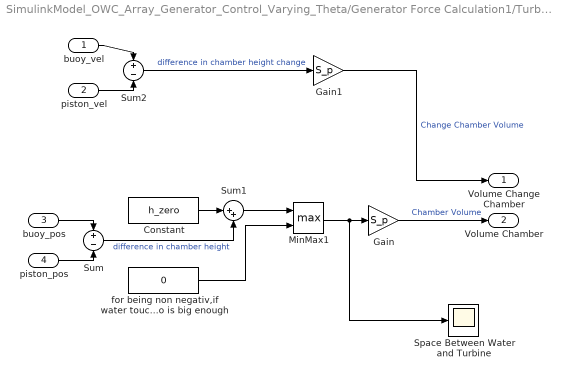
== system SimulinkModel_OWC_Array_Generator_Control_Varying_Theta/Generator Force Calculation1/Turbine//Generator Dynamics/Subsystem1/Chamber  ==
  buoy_vel : Inport
  piston_vel : Inport  Port=2
  buoy_pos : Inport  Port=3
  "piston_pos " : Inport  Port=4
  Constant : Constant  Value=h_zero
  Gain : Gain  Gain=S_p
  Gain1 : Gain  Gain=S_p
  MinMax1 : MinMax  Function=max  Inputs=2
  Space Between Water and Turbine : Scope
  Sum : Sum  Inputs=+-
  Sum1 : Sum  Inputs=|++
  Sum2 : Sum  Inputs=+-
  for being non negativ,if water touches turbine error will occur. usually not the case if h_zero is big enough : Constant  Value=0
  "Volume Change Chamber " : Outport
  Volume Chamber : Outport  Port=2
  wires:
  MinMax1/1 -> Gain/1, Space Between Water and Turbine/1
  for being non negativ,if water touches turbine error will occur. usually not the case if h_zero is big enough/1 -> MinMax1/2
  Gain1/1 -> "Volume Change Chamber "/1  "Change Chamber Volume"
  Gain/1 -> Volume Chamber/1  "Chamber Volume"
  buoy_pos/1 -> Sum/1
  Constant/1 -> Sum1/1
  buoy_vel/1 -> Sum2/1
  Sum2/1 -> Gain1/1  "difference in chamber height change"
  Sum/1 -> Sum1/2  "difference in chamber height"
  "piston_pos "/1 -> Sum/2
  piston_vel/1 -> Sum2/2
  Sum1/1 -> MinMax1/1

== system SimulinkModel_OWC_Array_Generator_Control_Varying_Theta/Generator Force Calculation1/Turbine//Generator Dynamics/Subsystem1/p*^(y-1//y) ==
  In1 : Inport
  Demux3 : Demux  Outputs=3
  Fcn : Fcn  Expr=u^((gamma-1)/gamma)
  Fcn4 : Fcn  Expr=u^((gamma-1)/gamma)
  Fcn5 : Fcn  Expr=u^((gamma-1)/gamma)
  Mux3 : Mux  Inputs=3
  Out1 : Outport
  wires:
  In1/1 -> Demux3/1
  Fcn4/1 -> Mux3/1
  Fcn5/1 -> Mux3/3
  Mux3/1 -> Out1/1
  Demux3/2 -> Fcn/1
  Fcn/1 -> Mux3/2
  Demux3/1 -> Fcn4/1
  Demux3/3 -> Fcn5/1

== system SimulinkModel_OWC_Array_Generator_Control_Varying_Theta/Generator Force Calculation1/Turbine//Generator Dynamics/Generator Control/Subsystem/Subsystem ==
  input2 : Inport
  Demux1 : Demux  Outputs=3
  MinMax : MinMax  Function=max
  MinMax1 : MinMax  Function=max
  MinMax2 : MinMax  Function=max
  Mux1 : Mux  Inputs=3
  "max " : Outport
  wires:
  MinMax/1 -> Mux1/1
  Demux1/3 -> MinMax2/1
  Mux1/1 -> "max "/1
  MinMax2/1 -> Mux1/3
  Demux1/1 -> MinMax/1
  Demux1/2 -> MinMax1/1
  MinMax1/1 -> Mux1/2
  input2/1 -> Demux1/1

== system SimulinkModel_OWC_Array_Generator_Control_Varying_Theta/Generator Force Calculation1/Turbine//Generator Dynamics/Generator Control/Subsystem/square ==
  Omega : Inport
  Demux1 : Demux  Outputs=3
  Math Function4 : Math  Operator=square  SaturateOnIntegerOverflow=on
  Math Function5 : Math  Operator=square  SaturateOnIntegerOverflow=on
  Math Function6 : Math  Operator=square  SaturateOnIntegerOverflow=on
  Mux1 : Mux  Inputs=3
  "OmegaSquared " : Outport
  wires:
  Math Function5/1 -> Mux1/2
  Demux1/3 -> Math Function6/1
  Omega/1 -> Demux1/1
  Demux1/1 -> Math Function4/1
  Demux1/2 -> Math Function5/1
  Mux1/1 -> "OmegaSquared "/1
  Math Function4/1 -> Mux1/1
  Math Function6/1 -> Mux1/3

== matlab function SimulinkModel_OWC_Array_Generator_Control_Varying_Theta/Generator Force Calculation1/Turbine//Generator Dynamics/MATLAB Function ==
  data: pos input; y output; vel input; activate_HSSV input
function y = fcn(pos, vel,activate_HSSV)
P_HSSV = zeros(3,1);
if (activate_HSSV)
    for i = 4:6
        if abs(pos(i))>1.5 && abs(vel(i))<.4
            P_HSSV(i-3) = 1;
        end
    end
end
y = P_HSSV;

== matlab function SimulinkModel_OWC_Array_Generator_Control_Varying_Theta/Subsystem3/Check if user input equals irregular waves, then the special irregular excitation force, else the user input times the linear excitation force coeff ==
  data: userWaves input; y output; irregEta input; irregEx input; FEX input
function y = fcn(userWaves,irregEta,irregEx,FEX)
if userWaves == irregEta
    y = irregEx;
else
    y = userWaves.*FEX;
end
